simulink model "HW3Prob3"  (R2021a)
settings: Solver=VariableStepAuto  StartTime=0.0  StopTime=10.0  RelTol=1e-3
model workspace (MAT data in the model file):
  L = 1
  theta_dot = 1
  v = 1
  vL = 1
  vR = 1
  w = 1
settings Model: Creator=Jacob  LastModifiedBy=Jacob

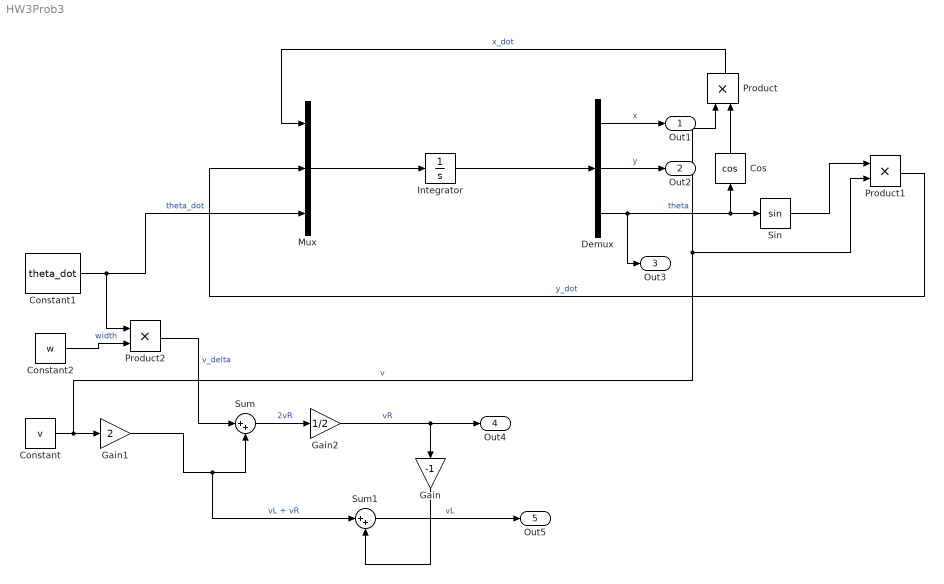
== system HW3Prob3 ==
  Constant : Constant  Value=v
  Constant1 : Constant  Value=theta_dot
  Constant2 : Constant  Value=w
  Cos : Trigonometry  Operator=cos
  Demux : Demux  Outputs=3
  Gain : Gain  Gain=-1
  Gain1 : Gain  Gain=2
  Gain2 : Gain  Gain=1/2
  Integrator : Integrator
  Mux : Mux  Inputs=3
  Product : Product
  Product1 : Product
  Product2 : Product
  Sin : Trigonometry
  Sum : Sum  Inputs=|++
  Sum1 : Sum  Inputs=|++
  Out1 : Outport
  Out2 : Outport  Port=2
  Out3 : Outport  Port=3
  Out4 : Outport  Port=4
  Out5 : Outport  Port=5
  wires:
  Product/1 -> Mux/1  "x_dot"
  Product1/1 -> Mux/2  "y_dot"
  Constant1/1 -> Product2/1, Mux/3  "theta_dot"
  Mux/1 -> Integrator/1
  Integrator/1 -> Demux/1
  Demux/3 -> Out3/1, Cos/1, Sin/1  "theta"
  Cos/1 -> Product/2
  Sin/1 -> Product1/1
  Demux/1 -> Out1/1  "x"
  Demux/2 -> Out2/1  "y"
  Constant2/1 -> Product2/2  "width"
  Product2/1 -> Sum/1  "v_delta"
  Constant/1 -> Product1/2, Product/1, Gain1/1  "v"
  Gain1/1 -> Sum1/1, Sum/2  "vL + vR"
  Sum/1 -> Gain2/1  "2vR"
  Gain2/1 -> Out4/1, Gain/1  "vR"
  Gain/1 -> Sum1/2
  Sum1/1 -> Out5/1  "vL"
